simulink model "REGISTROS_64_BITS_02"  (R2022a)
settings: Solver=VariableStepAuto  StartTime=0.0  StopTime=10.0  RelTol=1e-3
undefined symbols (not defined in the file or in its folder): xc7z010iclg225
libraries: hdlBasic x6609, vmcUtilities x1
(part 17 of 23)

== system REGISTROS_64_BITS_02/REGISTRO_64_BITS_8 ==
  D (64 BIT) : Inport
  C - ENABLE (1 BIT) : Inport  Port=2
  Concat1 : hdlBasic/Concat  num_inputs=2  XmcBlockStatus=1  maskContainerNames=group1  block_type=concat  block_config=sysgen:Concat_config
  Convert32 : hdlBasic/Convert  gui_display_data_type=Boolean  arith_type=Boolean  n_bits=16  bin_pt=14  float_type=Single  exp_bits=8  fraction_bits=24  quantization=Truncate  overflow=Wrap  en=off  latency=0  pipeline=off  XmcBlockStatus=1  maskContainerNames=group2  block_type=convert  block_config=sysgen:Convert_config  block_width=595  block_height=885
  D_0 : hdlBasic/Slice  nbits=1  boolean_output=off  mode=Lower Bit Location + Width  bit1=-3  base1=MSB of Input  bit0=0  base0=LSB of Input  XmcBlockStatus=1  maskContainerNames=group1  block_type=slice  block_config=sysgen:Slice_config
  D_1 : hdlBasic/Slice  nbits=1  boolean_output=off  mode=Lower Bit Location + Width  bit1=-2  base1=MSB of Input  bit0=1  base0=LSB of Input  XmcBlockStatus=1  maskContainerNames=group1  block_type=slice  block_config=sysgen:Slice_config
  D_10 : hdlBasic/Slice  nbits=1  boolean_output=off  mode=Lower Bit Location + Width  bit1=-1  base1=MSB of Input  bit0=10  base0=LSB of Input  XmcBlockStatus=1  maskContainerNames=group1  block_type=slice  block_config=sysgen:Slice_config
  D_11 : hdlBasic/Slice  nbits=1  boolean_output=off  mode=Lower Bit Location + Width  bit1=0  base1=MSB of Input  bit0=11  base0=LSB of Input  XmcBlockStatus=1  maskContainerNames=group1  block_type=slice  block_config=sysgen:Slice_config
  D_12 : hdlBasic/Slice  nbits=1  boolean_output=off  mode=Lower Bit Location + Width  bit1=-3  base1=MSB of Input  bit0=12  base0=LSB of Input  XmcBlockStatus=1  maskContainerNames=group1  block_type=slice  block_config=sysgen:Slice_config
  D_13 : hdlBasic/Slice  nbits=1  boolean_output=off  mode=Lower Bit Location + Width  bit1=-2  base1=MSB of Input  bit0=13  base0=LSB of Input  XmcBlockStatus=1  maskContainerNames=group1  block_type=slice  block_config=sysgen:Slice_config
  D_14 : hdlBasic/Slice  nbits=1  boolean_output=off  mode=Lower Bit Location + Width  bit1=-1  base1=MSB of Input  bit0=14  base0=LSB of Input  XmcBlockStatus=1  maskContainerNames=group1  block_type=slice  block_config=sysgen:Slice_config
  D_15 : hdlBasic/Slice  nbits=1  boolean_output=off  mode=Lower Bit Location + Width  bit1=0  base1=MSB of Input  bit0=15  base0=LSB of Input  XmcBlockStatus=1  maskContainerNames=group1  block_type=slice  block_config=sysgen:Slice_config
  D_16 : hdlBasic/Slice  nbits=1  boolean_output=off  mode=Lower Bit Location + Width  bit1=-3  base1=MSB of Input  bit0=16  base0=LSB of Input  XmcBlockStatus=1  maskContainerNames=group1  block_type=slice  block_config=sysgen:Slice_config
  D_17 : hdlBasic/Slice  nbits=1  boolean_output=off  mode=Lower Bit Location + Width  bit1=-2  base1=MSB of Input  bit0=17  base0=LSB of Input  XmcBlockStatus=1  maskContainerNames=group1  block_type=slice  block_config=sysgen:Slice_config
  D_18 : hdlBasic/Slice  nbits=1  boolean_output=off  mode=Lower Bit Location + Width  bit1=-1  base1=MSB of Input  bit0=18  base0=LSB of Input  XmcBlockStatus=1  maskContainerNames=group1  block_type=slice  block_config=sysgen:Slice_config
  D_19 : hdlBasic/Slice  nbits=1  boolean_output=off  mode=Lower Bit Location + Width  bit1=0  base1=MSB of Input  bit0=19  base0=LSB of Input  XmcBlockStatus=1  maskContainerNames=group1  block_type=slice  block_config=sysgen:Slice_config
  D_2 : hdlBasic/Slice  nbits=1  boolean_output=off  mode=Lower Bit Location + Width  bit1=-1  base1=MSB of Input  bit0=2  base0=LSB of Input  XmcBlockStatus=1  maskContainerNames=group1  block_type=slice  block_config=sysgen:Slice_config
  D_20 : hdlBasic/Slice  nbits=1  boolean_output=off  mode=Lower Bit Location + Width  bit1=-3  base1=MSB of Input  bit0=20  base0=LSB of Input  XmcBlockStatus=1  maskContainerNames=group1  block_type=slice  block_config=sysgen:Slice_config
  D_21 : hdlBasic/Slice  nbits=1  boolean_output=off  mode=Lower Bit Location + Width  bit1=-2  base1=MSB of Input  bit0=21  base0=LSB of Input  XmcBlockStatus=1  maskContainerNames=group1  block_type=slice  block_config=sysgen:Slice_config
  D_22 : hdlBasic/Slice  nbits=1  boolean_output=off  mode=Lower Bit Location + Width  bit1=-1  base1=MSB of Input  bit0=22  base0=LSB of Input  XmcBlockStatus=1  maskContainerNames=group1  block_type=slice  block_config=sysgen:Slice_config
  D_23 : hdlBasic/Slice  nbits=1  boolean_output=off  mode=Lower Bit Location + Width  bit1=0  base1=MSB of Input  bit0=23  base0=LSB of Input  XmcBlockStatus=1  maskContainerNames=group1  block_type=slice  block_config=sysgen:Slice_config
  D_24 : hdlBasic/Slice  nbits=1  boolean_output=off  mode=Lower Bit Location + Width  bit1=-3  base1=MSB of Input  bit0=24  base0=LSB of Input  XmcBlockStatus=1  maskContainerNames=group1  block_type=slice  block_config=sysgen:Slice_config
  D_25 : hdlBasic/Slice  nbits=1  boolean_output=off  mode=Lower Bit Location + Width  bit1=-2  base1=MSB of Input  bit0=25  base0=LSB of Input  XmcBlockStatus=1  maskContainerNames=group1  block_type=slice  block_config=sysgen:Slice_config
  D_26 : hdlBasic/Slice  nbits=1  boolean_output=off  mode=Lower Bit Location + Width  bit1=-1  base1=MSB of Input  bit0=26  base0=LSB of Input  XmcBlockStatus=1  maskContainerNames=group1  block_type=slice  block_config=sysgen:Slice_config
  D_27 : hdlBasic/Slice  nbits=1  boolean_output=off  mode=Lower Bit Location + Width  bit1=0  base1=MSB of Input  bit0=27  base0=LSB of Input  XmcBlockStatus=1  maskContainerNames=group1  block_type=slice  block_config=sysgen:Slice_config
  D_28 : hdlBasic/Slice  nbits=1  boolean_output=off  mode=Lower Bit Location + Width  bit1=-3  base1=MSB of Input  bit0=28  base0=LSB of Input  XmcBlockStatus=1  maskContainerNames=group1  block_type=slice  block_config=sysgen:Slice_config
  D_29 : hdlBasic/Slice  nbits=1  boolean_output=off  mode=Lower Bit Location + Width  bit1=-2  base1=MSB of Input  bit0=29  base0=LSB of Input  XmcBlockStatus=1  maskContainerNames=group1  block_type=slice  block_config=sysgen:Slice_config
  D_3 : hdlBasic/Slice  nbits=1  boolean_output=off  mode=Lower Bit Location + Width  bit1=0  base1=MSB of Input  bit0=3  base0=LSB of Input  XmcBlockStatus=1  maskContainerNames=group1  block_type=slice  block_config=sysgen:Slice_config
  D_30 : hdlBasic/Slice  nbits=1  boolean_output=off  mode=Lower Bit Location + Width  bit1=-1  base1=MSB of Input  bit0=30  base0=LSB of Input  XmcBlockStatus=1  maskContainerNames=group1  block_type=slice  block_config=sysgen:Slice_config
  D_31 : hdlBasic/Slice  nbits=1  boolean_output=off  mode=Lower Bit Location + Width  bit1=0  base1=MSB of Input  bit0=31  base0=LSB of Input  XmcBlockStatus=1  maskContainerNames=group1  block_type=slice  block_config=sysgen:Slice_config
  D_32 : hdlBasic/Slice  nbits=1  boolean_output=off  mode=Lower Bit Location + Width  bit1=-3  base1=MSB of Input  bit0=32  base0=LSB of Input  XmcBlockStatus=1  maskContainerNames=group1  block_type=slice  block_config=sysgen:Slice_config
  D_33 : hdlBasic/Slice  nbits=1  boolean_output=off  mode=Lower Bit Location + Width  bit1=-2  base1=MSB of Input  bit0=33  base0=LSB of Input  XmcBlockStatus=1  maskContainerNames=group1  block_type=slice  block_config=sysgen:Slice_config
  D_34 : hdlBasic/Slice  nbits=1  boolean_output=off  mode=Lower Bit Location + Width  bit1=-1  base1=MSB of Input  bit0=34  base0=LSB of Input  XmcBlockStatus=1  maskContainerNames=group1  block_type=slice  block_config=sysgen:Slice_config
  D_35 : hdlBasic/Slice  nbits=1  boolean_output=off  mode=Lower Bit Location + Width  bit1=0  base1=MSB of Input  bit0=35  base0=LSB of Input  XmcBlockStatus=1  maskContainerNames=group1  block_type=slice  block_config=sysgen:Slice_config
  D_36 : hdlBasic/Slice  nbits=1  boolean_output=off  mode=Lower Bit Location + Width  bit1=-3  base1=MSB of Input  bit0=36  base0=LSB of Input  XmcBlockStatus=1  maskContainerNames=group1  block_type=slice  block_config=sysgen:Slice_config
  D_37 : hdlBasic/Slice  nbits=1  boolean_output=off  mode=Lower Bit Location + Width  bit1=-2  base1=MSB of Input  bit0=37  base0=LSB of Input  XmcBlockStatus=1  maskContainerNames=group1  block_type=slice  block_config=sysgen:Slice_config
  D_38 : hdlBasic/Slice  nbits=1  boolean_output=off  mode=Lower Bit Location + Width  bit1=-1  base1=MSB of Input  bit0=38  base0=LSB of Input  XmcBlockStatus=1  maskContainerNames=group1  block_type=slice  block_config=sysgen:Slice_config
  D_39 : hdlBasic/Slice  nbits=1  boolean_output=off  mode=Lower Bit Location + Width  bit1=0  base1=MSB of Input  bit0=39  base0=LSB of Input  XmcBlockStatus=1  maskContainerNames=group1  block_type=slice  block_config=sysgen:Slice_config
  D_4 : hdlBasic/Slice  nbits=1  boolean_output=off  mode=Lower Bit Location + Width  bit1=-3  base1=MSB of Input  bit0=4  base0=LSB of Input  XmcBlockStatus=1  maskContainerNames=group1  block_type=slice  block_config=sysgen:Slice_config
  D_40 : hdlBasic/Slice  nbits=1  boolean_output=off  mode=Lower Bit Location + Width  bit1=-3  base1=MSB of Input  bit0=40  base0=LSB of Input  XmcBlockStatus=1  maskContainerNames=group1  block_type=slice  block_config=sysgen:Slice_config
  D_41 : hdlBasic/Slice  nbits=1  boolean_output=off  mode=Lower Bit Location + Width  bit1=-2  base1=MSB of Input  bit0=41  base0=LSB of Input  XmcBlockStatus=1  maskContainerNames=group1  block_type=slice  block_config=sysgen:Slice_config
  D_42 : hdlBasic/Slice  nbits=1  boolean_output=off  mode=Lower Bit Location + Width  bit1=-1  base1=MSB of Input  bit0=42  base0=LSB of Input  XmcBlockStatus=1  maskContainerNames=group1  block_type=slice  block_config=sysgen:Slice_config
  D_43 : hdlBasic/Slice  nbits=1  boolean_output=off  mode=Lower Bit Location + Width  bit1=0  base1=MSB of Input  bit0=43  base0=LSB of Input  XmcBlockStatus=1  maskContainerNames=group1  block_type=slice  block_config=sysgen:Slice_config
  D_44 : hdlBasic/Slice  nbits=1  boolean_output=off  mode=Lower Bit Location + Width  bit1=-3  base1=MSB of Input  bit0=44  base0=LSB of Input  XmcBlockStatus=1  maskContainerNames=group1  block_type=slice  block_config=sysgen:Slice_config
  D_45 : hdlBasic/Slice  nbits=1  boolean_output=off  mode=Lower Bit Location + Width  bit1=-2  base1=MSB of Input  bit0=45  base0=LSB of Input  XmcBlockStatus=1  maskContainerNames=group1  block_type=slice  block_config=sysgen:Slice_config
  D_46 : hdlBasic/Slice  nbits=1  boolean_output=off  mode=Lower Bit Location + Width  bit1=-1  base1=MSB of Input  bit0=46  base0=LSB of Input  XmcBlockStatus=1  maskContainerNames=group1  block_type=slice  block_config=sysgen:Slice_config
  D_47 : hdlBasic/Slice  nbits=1  boolean_output=off  mode=Lower Bit Location + Width  bit1=0  base1=MSB of Input  bit0=47  base0=LSB of Input  XmcBlockStatus=1  maskContainerNames=group1  block_type=slice  block_config=sysgen:Slice_config
  D_48 : hdlBasic/Slice  nbits=1  boolean_output=off  mode=Lower Bit Location + Width  bit1=-3  base1=MSB of Input  bit0=48  base0=LSB of Input  XmcBlockStatus=1  maskContainerNames=group1  block_type=slice  block_config=sysgen:Slice_config
  D_49 : hdlBasic/Slice  nbits=1  boolean_output=off  mode=Lower Bit Location + Width  bit1=-2  base1=MSB of Input  bit0=49  base0=LSB of Input  XmcBlockStatus=1  maskContainerNames=group1  block_type=slice  block_config=sysgen:Slice_config
  D_5 : hdlBasic/Slice  nbits=1  boolean_output=off  mode=Lower Bit Location + Width  bit1=-2  base1=MSB of Input  bit0=5  base0=LSB of Input  XmcBlockStatus=1  maskContainerNames=group1  block_type=slice  block_config=sysgen:Slice_config
  D_50 : hdlBasic/Slice  nbits=1  boolean_output=off  mode=Lower Bit Location + Width  bit1=-1  base1=MSB of Input  bit0=50  base0=LSB of Input  XmcBlockStatus=1  maskContainerNames=group1  block_type=slice  block_config=sysgen:Slice_config
  D_51 : hdlBasic/Slice  nbits=1  boolean_output=off  mode=Lower Bit Location + Width  bit1=0  base1=MSB of Input  bit0=51  base0=LSB of Input  XmcBlockStatus=1  maskContainerNames=group1  block_type=slice  block_config=sysgen:Slice_config
  D_52 : hdlBasic/Slice  nbits=1  boolean_output=off  mode=Lower Bit Location + Width  bit1=-3  base1=MSB of Input  bit0=52  base0=LSB of Input  XmcBlockStatus=1  maskContainerNames=group1  block_type=slice  block_config=sysgen:Slice_config
  D_53 : hdlBasic/Slice  nbits=1  boolean_output=off  mode=Lower Bit Location + Width  bit1=-2  base1=MSB of Input  bit0=53  base0=LSB of Input  XmcBlockStatus=1  maskContainerNames=group1  block_type=slice  block_config=sysgen:Slice_config
  D_54 : hdlBasic/Slice  nbits=1  boolean_output=off  mode=Lower Bit Location + Width  bit1=-1  base1=MSB of Input  bit0=54  base0=LSB of Input  XmcBlockStatus=1  maskContainerNames=group1  block_type=slice  block_config=sysgen:Slice_config
  D_55 : hdlBasic/Slice  nbits=1  boolean_output=off  mode=Lower Bit Location + Width  bit1=0  base1=MSB of Input  bit0=55  base0=LSB of Input  XmcBlockStatus=1  maskContainerNames=group1  block_type=slice  block_config=sysgen:Slice_config
  D_56 : hdlBasic/Slice  nbits=1  boolean_output=off  mode=Lower Bit Location + Width  bit1=-3  base1=MSB of Input  bit0=56  base0=LSB of Input  XmcBlockStatus=1  maskContainerNames=group1  block_type=slice  block_config=sysgen:Slice_config
  D_57 : hdlBasic/Slice  nbits=1  boolean_output=off  mode=Lower Bit Location + Width  bit1=-2  base1=MSB of Input  bit0=57  base0=LSB of Input  XmcBlockStatus=1  maskContainerNames=group1  block_type=slice  block_config=sysgen:Slice_config
  D_58 : hdlBasic/Slice  nbits=1  boolean_output=off  mode=Lower Bit Location + Width  bit1=-1  base1=MSB of Input  bit0=58  base0=LSB of Input  XmcBlockStatus=1  maskContainerNames=group1  block_type=slice  block_config=sysgen:Slice_config
  D_59 : hdlBasic/Slice  nbits=1  boolean_output=off  mode=Lower Bit Location + Width  bit1=0  base1=MSB of Input  bit0=59  base0=LSB of Input  XmcBlockStatus=1  maskContainerNames=group1  block_type=slice  block_config=sysgen:Slice_config
  D_6 : hdlBasic/Slice  nbits=1  boolean_output=off  mode=Lower Bit Location + Width  bit1=-1  base1=MSB of Input  bit0=6  base0=LSB of Input  XmcBlockStatus=1  maskContainerNames=group1  block_type=slice  block_config=sysgen:Slice_config
  D_60 : hdlBasic/Slice  nbits=1  boolean_output=off  mode=Lower Bit Location + Width  bit1=-3  base1=MSB of Input  bit0=60  base0=LSB of Input  XmcBlockStatus=1  maskContainerNames=group1  block_type=slice  block_config=sysgen:Slice_config
  D_61 : hdlBasic/Slice  nbits=1  boolean_output=off  mode=Lower Bit Location + Width  bit1=-2  base1=MSB of Input  bit0=61  base0=LSB of Input  XmcBlockStatus=1  maskContainerNames=group1  block_type=slice  block_config=sysgen:Slice_config
  D_62 : hdlBasic/Slice  nbits=1  boolean_output=off  mode=Lower Bit Location + Width  bit1=-1  base1=MSB of Input  bit0=62  base0=LSB of Input  XmcBlockStatus=1  maskContainerNames=group1  block_type=slice  block_config=sysgen:Slice_config
  D_63 : hdlBasic/Slice  nbits=1  boolean_output=off  mode=Lower Bit Location + Width  bit1=0  base1=MSB of Input  bit0=63  base0=LSB of Input  XmcBlockStatus=1  maskContainerNames=group1  block_type=slice  block_config=sysgen:Slice_config
  D_7 : hdlBasic/Slice  nbits=1  boolean_output=off  mode=Lower Bit Location + Width  bit1=0  base1=MSB of Input  bit0=7  base0=LSB of Input  XmcBlockStatus=1  maskContainerNames=group1  block_type=slice  block_config=sysgen:Slice_config
  D_8 : hdlBasic/Slice  nbits=1  boolean_output=off  mode=Lower Bit Location + Width  bit1=-3  base1=MSB of Input  bit0=8  base0=LSB of Input  XmcBlockStatus=1  maskContainerNames=group1  block_type=slice  block_config=sysgen:Slice_config
  D_9 : hdlBasic/Slice  nbits=1  boolean_output=off  mode=Lower Bit Location + Width  bit1=-2  base1=MSB of Input  bit0=9  base0=LSB of Input  XmcBlockStatus=1  maskContainerNames=group1  block_type=slice  block_config=sysgen:Slice_config
  Q_OUT_32_BIT1 : Subsystem
  Q_OUT_32_BIT2 : Subsystem
  Register_{1..64} (64 alike) : hdlBasic/Register  init=0  rst=off  en=on  XmcBlockStatus=1  maskContainerNames=tabcontainer1  block_type=register  block_config=sysgen:Register_config
  Q (64 BIT) : Outport
  wires:
  D (64 BIT)/1 -> D_63/1, D_62/1, D_61/1, D_60/1, D_59/1, D_58/1, D_57/1, D_56/1, D_55/1, D_54/1, D_53/1, D_52/1, D_51/1, D_50/1, D_49/1, D_48/1, D_47/1, D_46/1, D_45/1, D_44/1, D_43/1, D_42/1, D_41/1, D_40/1, D_39/1, D_38/1, D_37/1, D_36/1, D_35/1, D_34/1, D_33/1, D_32/1, D_31/1, D_30/1, D_29/1, D_28/1, D_27/1, D_26/1, D_25/1, D_24/1, D_23/1, D_22/1, D_21/1, D_20/1, D_19/1, D_18/1, D_17/1, D_16/1, D_15/1, D_14/1, D_13/1, D_12/1, D_11/1, D_10/1, D_9/1, D_8/1, D_7/1, D_6/1, D_5/1, D_4/1, D_3/1, D_2/1, D_1/1, D_0/1
  Register_27/1 -> Q_OUT_32_BIT2/27(Q_OUT_26 (1 BIT))
  D_59/1 -> Register_28/1
  Register_4/1 -> Q_OUT_32_BIT2/4(Q_OUT_3 (1 BIT))
  Register_21/1 -> Q_OUT_32_BIT2/21(Q_OUT_20 (1 BIT))
  Register_56/1 -> Q_OUT_32_BIT1/25(Q_OUT_24 (1 BIT))
  C - ENABLE (1 BIT)/1 -> Convert32/1
  Register_3/1 -> Q_OUT_32_BIT2/3(Q_OUT_2 (1 BIT))
  D_19/1 -> Register_51/1
  D_12/1 -> Register_44/1
  Convert32/1 -> Register_35/2, Register_49/2, Register_64/2, Register_31/2, Register_30/2, Register_29/2, Register_28/2, Register_27/2, Register_26/2, Register_25/2, Register_24/2, Register_23/2, Register_22/2, Register_21/2, Register_20/2, Register_19/2, Register_18/2, Register_17/2, Register_16/2, Register_15/2, Register_14/2, Register_13/2, Register_12/2, Register_11/2, Register_10/2, Register_9/2, Register_8/2, Register_7/2, Register_6/2, Register_5/2, Register_4/2, Register_3/2, Register_2/2, Register_1/2, Register_63/2, Register_62/2, Register_61/2, Register_60/2, Register_59/2, Register_58/2, Register_57/2, Register_56/2, Register_55/2, Register_54/2, Register_53/2, Register_52/2, Register_51/2, Register_50/2, Register_48/2, Register_47/2, Register_46/2, Register_45/2, Register_44/2, Register_43/2, Register_42/2, Register_41/2, Register_40/2, Register_39/2, Register_38/2, Register_37/2, Register_36/2, Register_34/2, Register_33/2, Register_32/2
  D_2/1 -> Register_34/1
  Register_49/1 -> Q_OUT_32_BIT1/18(Q_OUT_17 (1 BIT))
  D_37/1 -> Register_6/1
  D_3/1 -> Register_35/1
  Register_8/1 -> Q_OUT_32_BIT2/8(Q_OUT_7 (1 BIT))
  D_47/1 -> Register_16/1
  Register_34/1 -> Q_OUT_32_BIT1/3(Q_OUT_2 (1 BIT))
  D_29/1 -> Register_61/1
  Register_26/1 -> Q_OUT_32_BIT2/26(Q_OUT_25 (1 BIT))
  D_6/1 -> Register_38/1
  Register_40/1 -> Q_OUT_32_BIT1/9(Q_OUT_8 (1 BIT))
  D_17/1 -> Register_49/1
  Register_9/1 -> Q_OUT_32_BIT2/9(Q_OUT_8 (1 BIT))
  Register_61/1 -> Q_OUT_32_BIT1/30(Q_OUT_29 (1 BIT))
  D_49/1 -> Register_18/1
  D_32/1 -> Register_1/1
  D_10/1 -> Register_42/1
  Register_62/1 -> Q_OUT_32_BIT1/31(Q_OUT_30 (1 BIT))
  D_18/1 -> Register_50/1
  Register_11/1 -> Q_OUT_32_BIT2/11(Q_OUT_10 (1 BIT))
  D_61/1 -> Register_30/1
  D_16/1 -> Register_48/1
  D_56/1 -> Register_25/1
  Register_30/1 -> Q_OUT_32_BIT2/30(Q_OUT_29 (1 BIT))
  Register_23/1 -> Q_OUT_32_BIT2/23(Q_OUT_22 (1 BIT))
  Concat1/1 -> Q (64 BIT)/1
  D_27/1 -> Register_59/1
  D_1/1 -> Register_33/1
  Register_60/1 -> Q_OUT_32_BIT1/29(Q_OUT_28 (1 BIT))
  Register_59/1 -> Q_OUT_32_BIT1/28(Q_OUT_27 (1 BIT))
  Register_33/1 -> Q_OUT_32_BIT1/2(Q_OUT_1 (1 BIT))
  Register_1/1 -> Q_OUT_32_BIT2/1(Q_OUT_0 (1 BIT))
  Register_5/1 -> Q_OUT_32_BIT2/5(Q_OUT_4 (1 BIT))
  Register_48/1 -> Q_OUT_32_BIT1/17(Q_OUT_16 (1 BIT))
  Register_53/1 -> Q_OUT_32_BIT1/22(Q_OUT_21 (1 BIT))
  D_58/1 -> Register_27/1
  Register_15/1 -> Q_OUT_32_BIT2/15(Q_OUT_14 (1 BIT))
  Register_35/1 -> Q_OUT_32_BIT1/4(Q_OUT_3 (1 BIT))
  D_26/1 -> Register_58/1
  D_22/1 -> Register_54/1
  D_4/1 -> Register_36/1
  D_0/1 -> Register_32/1
  D_23/1 -> Register_55/1
  Register_38/1 -> Q_OUT_32_BIT1/7(Q_OUT_6 (1 BIT))
  D_25/1 -> Register_57/1
  Register_24/1 -> Q_OUT_32_BIT2/24(Q_OUT_23 (1 BIT))
  Register_55/1 -> Q_OUT_32_BIT1/24(Q_OUT_23 (1 BIT))
  Register_16/1 -> Q_OUT_32_BIT2/16(Q_OUT_15 (1 BIT))
  Register_51/1 -> Q_OUT_32_BIT1/20(Q_OUT_19 (1 BIT))
  Register_39/1 -> Q_OUT_32_BIT1/8(Q_OUT_7 (1 BIT))
  Register_42/1 -> Q_OUT_32_BIT1/11(Q_OUT_10 (1 BIT))
  D_38/1 -> Register_7/1
  Register_25/1 -> Q_OUT_32_BIT2/25(Q_OUT_24 (1 BIT))
  D_30/1 -> Register_62/1
  D_53/1 -> Register_22/1
  D_5/1 -> Register_37/1
  D_8/1 -> Register_40/1
  D_11/1 -> Register_43/1
  Register_57/1 -> Q_OUT_32_BIT1/26(Q_OUT_25 (1 BIT))
  Register_54/1 -> Q_OUT_32_BIT1/23(Q_OUT_22 (1 BIT))
  Register_50/1 -> Q_OUT_32_BIT1/19(Q_OUT_18 (1 BIT))
  Register_52/1 -> Q_OUT_32_BIT1/21(Q_OUT_20 (1 BIT))
  Register_44/1 -> Q_OUT_32_BIT1/13(Q_OUT_12 (1 BIT))
  Register_6/1 -> Q_OUT_32_BIT2/6(Q_OUT_5 (1 BIT))
  Register_13/1 -> Q_OUT_32_BIT2/13(Q_OUT_12 (1 BIT))
  D_42/1 -> Register_11/1
  Register_45/1 -> Q_OUT_32_BIT1/14(Q_OUT_13 (1 BIT))
  Register_58/1 -> Q_OUT_32_BIT1/27(Q_OUT_26 (1 BIT))
  Register_64/1 -> Q_OUT_32_BIT2/32(Q_OUT_31 (1 BIT))
  Register_2/1 -> Q_OUT_32_BIT2/2(Q_OUT_1 (1 BIT))
  Register_18/1 -> Q_OUT_32_BIT2/18(Q_OUT_17 (1 BIT))
  Register_31/1 -> Q_OUT_32_BIT2/31(Q_OUT_30 (1 BIT))
  Register_29/1 -> Q_OUT_32_BIT2/29(Q_OUT_28 (1 BIT))
  Register_12/1 -> Q_OUT_32_BIT2/12(Q_OUT_11 (1 BIT))
  Register_14/1 -> Q_OUT_32_BIT2/14(Q_OUT_13 (1 BIT))
  Register_36/1 -> Q_OUT_32_BIT1/5(Q_OUT_4 (1 BIT))
  Register_47/1 -> Q_OUT_32_BIT1/16(Q_OUT_15 (1 BIT))
  Register_41/1 -> Q_OUT_32_BIT1/10(Q_OUT_9 (1 BIT))
  Register_46/1 -> Q_OUT_32_BIT1/15(Q_OUT_14 (1 BIT))
  Register_32/1 -> Q_OUT_32_BIT1/1(Q_OUT_0 (1 BIT))
  D_28/1 -> Register_60/1
  Q_OUT_32_BIT2/1(Q (32 BIT)) -> Concat1/1
  Q_OUT_32_BIT1/1(Q (32 BIT)) -> Concat1/2
  D_43/1 -> Register_12/1
  D_57/1 -> Register_26/1
  D_63/1 -> Register_64/1
  D_45/1 -> Register_14/1
  D_46/1 -> Register_15/1
  D_39/1 -> Register_8/1
  D_52/1 -> Register_21/1
  D_41/1 -> Register_10/1
  D_60/1 -> Register_29/1
  D_35/1 -> Register_4/1
  D_54/1 -> Register_23/1
  D_62/1 -> Register_31/1
  D_15/1 -> Register_47/1
  D_48/1 -> Register_17/1
  D_40/1 -> Register_9/1
  D_7/1 -> Register_39/1
  D_36/1 -> Register_5/1
  D_55/1 -> Register_24/1
  D_51/1 -> Register_20/1
  D_44/1 -> Register_13/1
  D_34/1 -> Register_3/1
  D_33/1 -> Register_2/1
  D_50/1 -> Register_19/1
  D_9/1 -> Register_41/1
  Register_28/1 -> Q_OUT_32_BIT2/28(Q_OUT_27 (1 BIT))
  D_14/1 -> Register_46/1
  Register_7/1 -> Q_OUT_32_BIT2/7(Q_OUT_6 (1 BIT))
  Register_10/1 -> Q_OUT_32_BIT2/10(Q_OUT_9 (1 BIT))
  D_13/1 -> Register_45/1
  D_24/1 -> Register_56/1
  D_31/1 -> Register_63/1
  D_20/1 -> Register_52/1
  D_21/1 -> Register_53/1
  Register_63/1 -> Q_OUT_32_BIT1/32(Q_OUT_31 (1 BIT))
  Register_37/1 -> Q_OUT_32_BIT1/6(Q_OUT_5 (1 BIT))
  Register_20/1 -> Q_OUT_32_BIT2/20(Q_OUT_19 (1 BIT))
  Register_22/1 -> Q_OUT_32_BIT2/22(Q_OUT_21 (1 BIT))
  Register_19/1 -> Q_OUT_32_BIT2/19(Q_OUT_18 (1 BIT))
  Register_17/1 -> Q_OUT_32_BIT2/17(Q_OUT_16 (1 BIT))
  Register_43/1 -> Q_OUT_32_BIT1/12(Q_OUT_11 (1 BIT))

== system REGISTROS_64_BITS_02/REGISTRO_64_BITS_9 ==
  D (64 BIT) : Inport
  C - ENABLE (1 BIT) : Inport  Port=2
  Concat1 : hdlBasic/Concat  num_inputs=2  XmcBlockStatus=1  maskContainerNames=group1  block_type=concat  block_config=sysgen:Concat_config
  Convert32 : hdlBasic/Convert  gui_display_data_type=Boolean  arith_type=Boolean  n_bits=16  bin_pt=14  float_type=Single  exp_bits=8  fraction_bits=24  quantization=Truncate  overflow=Wrap  en=off  latency=0  pipeline=off  XmcBlockStatus=1  maskContainerNames=group2  block_type=convert  block_config=sysgen:Convert_config  block_width=595  block_height=885
  D_0 : hdlBasic/Slice  nbits=1  boolean_output=off  mode=Lower Bit Location + Width  bit1=-3  base1=MSB of Input  bit0=0  base0=LSB of Input  XmcBlockStatus=1  maskContainerNames=group1  block_type=slice  block_config=sysgen:Slice_config
  D_1 : hdlBasic/Slice  nbits=1  boolean_output=off  mode=Lower Bit Location + Width  bit1=-2  base1=MSB of Input  bit0=1  base0=LSB of Input  XmcBlockStatus=1  maskContainerNames=group1  block_type=slice  block_config=sysgen:Slice_config
  D_10 : hdlBasic/Slice  nbits=1  boolean_output=off  mode=Lower Bit Location + Width  bit1=-1  base1=MSB of Input  bit0=10  base0=LSB of Input  XmcBlockStatus=1  maskContainerNames=group1  block_type=slice  block_config=sysgen:Slice_config
  D_11 : hdlBasic/Slice  nbits=1  boolean_output=off  mode=Lower Bit Location + Width  bit1=0  base1=MSB of Input  bit0=11  base0=LSB of Input  XmcBlockStatus=1  maskContainerNames=group1  block_type=slice  block_config=sysgen:Slice_config
  D_12 : hdlBasic/Slice  nbits=1  boolean_output=off  mode=Lower Bit Location + Width  bit1=-3  base1=MSB of Input  bit0=12  base0=LSB of Input  XmcBlockStatus=1  maskContainerNames=group1  block_type=slice  block_config=sysgen:Slice_config
  D_13 : hdlBasic/Slice  nbits=1  boolean_output=off  mode=Lower Bit Location + Width  bit1=-2  base1=MSB of Input  bit0=13  base0=LSB of Input  XmcBlockStatus=1  maskContainerNames=group1  block_type=slice  block_config=sysgen:Slice_config
  D_14 : hdlBasic/Slice  nbits=1  boolean_output=off  mode=Lower Bit Location + Width  bit1=-1  base1=MSB of Input  bit0=14  base0=LSB of Input  XmcBlockStatus=1  maskContainerNames=group1  block_type=slice  block_config=sysgen:Slice_config
  D_15 : hdlBasic/Slice  nbits=1  boolean_output=off  mode=Lower Bit Location + Width  bit1=0  base1=MSB of Input  bit0=15  base0=LSB of Input  XmcBlockStatus=1  maskContainerNames=group1  block_type=slice  block_config=sysgen:Slice_config
  D_16 : hdlBasic/Slice  nbits=1  boolean_output=off  mode=Lower Bit Location + Width  bit1=-3  base1=MSB of Input  bit0=16  base0=LSB of Input  XmcBlockStatus=1  maskContainerNames=group1  block_type=slice  block_config=sysgen:Slice_config
  D_17 : hdlBasic/Slice  nbits=1  boolean_output=off  mode=Lower Bit Location + Width  bit1=-2  base1=MSB of Input  bit0=17  base0=LSB of Input  XmcBlockStatus=1  maskContainerNames=group1  block_type=slice  block_config=sysgen:Slice_config
  D_18 : hdlBasic/Slice  nbits=1  boolean_output=off  mode=Lower Bit Location + Width  bit1=-1  base1=MSB of Input  bit0=18  base0=LSB of Input  XmcBlockStatus=1  maskContainerNames=group1  block_type=slice  block_config=sysgen:Slice_config
  D_19 : hdlBasic/Slice  nbits=1  boolean_output=off  mode=Lower Bit Location + Width  bit1=0  base1=MSB of Input  bit0=19  base0=LSB of Input  XmcBlockStatus=1  maskContainerNames=group1  block_type=slice  block_config=sysgen:Slice_config
  D_2 : hdlBasic/Slice  nbits=1  boolean_output=off  mode=Lower Bit Location + Width  bit1=-1  base1=MSB of Input  bit0=2  base0=LSB of Input  XmcBlockStatus=1  maskContainerNames=group1  block_type=slice  block_config=sysgen:Slice_config
  D_20 : hdlBasic/Slice  nbits=1  boolean_output=off  mode=Lower Bit Location + Width  bit1=-3  base1=MSB of Input  bit0=20  base0=LSB of Input  XmcBlockStatus=1  maskContainerNames=group1  block_type=slice  block_config=sysgen:Slice_config
  D_21 : hdlBasic/Slice  nbits=1  boolean_output=off  mode=Lower Bit Location + Width  bit1=-2  base1=MSB of Input  bit0=21  base0=LSB of Input  XmcBlockStatus=1  maskContainerNames=group1  block_type=slice  block_config=sysgen:Slice_config
  D_22 : hdlBasic/Slice  nbits=1  boolean_output=off  mode=Lower Bit Location + Width  bit1=-1  base1=MSB of Input  bit0=22  base0=LSB of Input  XmcBlockStatus=1  maskContainerNames=group1  block_type=slice  block_config=sysgen:Slice_config
  D_23 : hdlBasic/Slice  nbits=1  boolean_output=off  mode=Lower Bit Location + Width  bit1=0  base1=MSB of Input  bit0=23  base0=LSB of Input  XmcBlockStatus=1  maskContainerNames=group1  block_type=slice  block_config=sysgen:Slice_config
  D_24 : hdlBasic/Slice  nbits=1  boolean_output=off  mode=Lower Bit Location + Width  bit1=-3  base1=MSB of Input  bit0=24  base0=LSB of Input  XmcBlockStatus=1  maskContainerNames=group1  block_type=slice  block_config=sysgen:Slice_config
  D_25 : hdlBasic/Slice  nbits=1  boolean_output=off  mode=Lower Bit Location + Width  bit1=-2  base1=MSB of Input  bit0=25  base0=LSB of Input  XmcBlockStatus=1  maskContainerNames=group1  block_type=slice  block_config=sysgen:Slice_config
  D_26 : hdlBasic/Slice  nbits=1  boolean_output=off  mode=Lower Bit Location + Width  bit1=-1  base1=MSB of Input  bit0=26  base0=LSB of Input  XmcBlockStatus=1  maskContainerNames=group1  block_type=slice  block_config=sysgen:Slice_config
  D_27 : hdlBasic/Slice  nbits=1  boolean_output=off  mode=Lower Bit Location + Width  bit1=0  base1=MSB of Input  bit0=27  base0=LSB of Input  XmcBlockStatus=1  maskContainerNames=group1  block_type=slice  block_config=sysgen:Slice_config
  D_28 : hdlBasic/Slice  nbits=1  boolean_output=off  mode=Lower Bit Location + Width  bit1=-3  base1=MSB of Input  bit0=28  base0=LSB of Input  XmcBlockStatus=1  maskContainerNames=group1  block_type=slice  block_config=sysgen:Slice_config
  D_29 : hdlBasic/Slice  nbits=1  boolean_output=off  mode=Lower Bit Location + Width  bit1=-2  base1=MSB of Input  bit0=29  base0=LSB of Input  XmcBlockStatus=1  maskContainerNames=group1  block_type=slice  block_config=sysgen:Slice_config
  D_3 : hdlBasic/Slice  nbits=1  boolean_output=off  mode=Lower Bit Location + Width  bit1=0  base1=MSB of Input  bit0=3  base0=LSB of Input  XmcBlockStatus=1  maskContainerNames=group1  block_type=slice  block_config=sysgen:Slice_config
  D_30 : hdlBasic/Slice  nbits=1  boolean_output=off  mode=Lower Bit Location + Width  bit1=-1  base1=MSB of Input  bit0=30  base0=LSB of Input  XmcBlockStatus=1  maskContainerNames=group1  block_type=slice  block_config=sysgen:Slice_config
  D_31 : hdlBasic/Slice  nbits=1  boolean_output=off  mode=Lower Bit Location + Width  bit1=0  base1=MSB of Input  bit0=31  base0=LSB of Input  XmcBlockStatus=1  maskContainerNames=group1  block_type=slice  block_config=sysgen:Slice_config
  D_32 : hdlBasic/Slice  nbits=1  boolean_output=off  mode=Lower Bit Location + Width  bit1=-3  base1=MSB of Input  bit0=32  base0=LSB of Input  XmcBlockStatus=1  maskContainerNames=group1  block_type=slice  block_config=sysgen:Slice_config
  D_33 : hdlBasic/Slice  nbits=1  boolean_output=off  mode=Lower Bit Location + Width  bit1=-2  base1=MSB of Input  bit0=33  base0=LSB of Input  XmcBlockStatus=1  maskContainerNames=group1  block_type=slice  block_config=sysgen:Slice_config
  D_34 : hdlBasic/Slice  nbits=1  boolean_output=off  mode=Lower Bit Location + Width  bit1=-1  base1=MSB of Input  bit0=34  base0=LSB of Input  XmcBlockStatus=1  maskContainerNames=group1  block_type=slice  block_config=sysgen:Slice_config
  D_35 : hdlBasic/Slice  nbits=1  boolean_output=off  mode=Lower Bit Location + Width  bit1=0  base1=MSB of Input  bit0=35  base0=LSB of Input  XmcBlockStatus=1  maskContainerNames=group1  block_type=slice  block_config=sysgen:Slice_config
  D_36 : hdlBasic/Slice  nbits=1  boolean_output=off  mode=Lower Bit Location + Width  bit1=-3  base1=MSB of Input  bit0=36  base0=LSB of Input  XmcBlockStatus=1  maskContainerNames=group1  block_type=slice  block_config=sysgen:Slice_config
  D_37 : hdlBasic/Slice  nbits=1  boolean_output=off  mode=Lower Bit Location + Width  bit1=-2  base1=MSB of Input  bit0=37  base0=LSB of Input  XmcBlockStatus=1  maskContainerNames=group1  block_type=slice  block_config=sysgen:Slice_config
  D_38 : hdlBasic/Slice  nbits=1  boolean_output=off  mode=Lower Bit Location + Width  bit1=-1  base1=MSB of Input  bit0=38  base0=LSB of Input  XmcBlockStatus=1  maskContainerNames=group1  block_type=slice  block_config=sysgen:Slice_config
  D_39 : hdlBasic/Slice  nbits=1  boolean_output=off  mode=Lower Bit Location + Width  bit1=0  base1=MSB of Input  bit0=39  base0=LSB of Input  XmcBlockStatus=1  maskContainerNames=group1  block_type=slice  block_config=sysgen:Slice_config
  D_4 : hdlBasic/Slice  nbits=1  boolean_output=off  mode=Lower Bit Location + Width  bit1=-3  base1=MSB of Input  bit0=4  base0=LSB of Input  XmcBlockStatus=1  maskContainerNames=group1  block_type=slice  block_config=sysgen:Slice_config
  D_40 : hdlBasic/Slice  nbits=1  boolean_output=off  mode=Lower Bit Location + Width  bit1=-3  base1=MSB of Input  bit0=40  base0=LSB of Input  XmcBlockStatus=1  maskContainerNames=group1  block_type=slice  block_config=sysgen:Slice_config
  D_41 : hdlBasic/Slice  nbits=1  boolean_output=off  mode=Lower Bit Location + Width  bit1=-2  base1=MSB of Input  bit0=41  base0=LSB of Input  XmcBlockStatus=1  maskContainerNames=group1  block_type=slice  block_config=sysgen:Slice_config
  D_42 : hdlBasic/Slice  nbits=1  boolean_output=off  mode=Lower Bit Location + Width  bit1=-1  base1=MSB of Input  bit0=42  base0=LSB of Input  XmcBlockStatus=1  maskContainerNames=group1  block_type=slice  block_config=sysgen:Slice_config
  D_43 : hdlBasic/Slice  nbits=1  boolean_output=off  mode=Lower Bit Location + Width  bit1=0  base1=MSB of Input  bit0=43  base0=LSB of Input  XmcBlockStatus=1  maskContainerNames=group1  block_type=slice  block_config=sysgen:Slice_config
  D_44 : hdlBasic/Slice  nbits=1  boolean_output=off  mode=Lower Bit Location + Width  bit1=-3  base1=MSB of Input  bit0=44  base0=LSB of Input  XmcBlockStatus=1  maskContainerNames=group1  block_type=slice  block_config=sysgen:Slice_config
  D_45 : hdlBasic/Slice  nbits=1  boolean_output=off  mode=Lower Bit Location + Width  bit1=-2  base1=MSB of Input  bit0=45  base0=LSB of Input  XmcBlockStatus=1  maskContainerNames=group1  block_type=slice  block_config=sysgen:Slice_config
  D_46 : hdlBasic/Slice  nbits=1  boolean_output=off  mode=Lower Bit Location + Width  bit1=-1  base1=MSB of Input  bit0=46  base0=LSB of Input  XmcBlockStatus=1  maskContainerNames=group1  block_type=slice  block_config=sysgen:Slice_config
  D_47 : hdlBasic/Slice  nbits=1  boolean_output=off  mode=Lower Bit Location + Width  bit1=0  base1=MSB of Input  bit0=47  base0=LSB of Input  XmcBlockStatus=1  maskContainerNames=group1  block_type=slice  block_config=sysgen:Slice_config
  D_48 : hdlBasic/Slice  nbits=1  boolean_output=off  mode=Lower Bit Location + Width  bit1=-3  base1=MSB of Input  bit0=48  base0=LSB of Input  XmcBlockStatus=1  maskContainerNames=group1  block_type=slice  block_config=sysgen:Slice_config
  D_49 : hdlBasic/Slice  nbits=1  boolean_output=off  mode=Lower Bit Location + Width  bit1=-2  base1=MSB of Input  bit0=49  base0=LSB of Input  XmcBlockStatus=1  maskContainerNames=group1  block_type=slice  block_config=sysgen:Slice_config
  D_5 : hdlBasic/Slice  nbits=1  boolean_output=off  mode=Lower Bit Location + Width  bit1=-2  base1=MSB of Input  bit0=5  base0=LSB of Input  XmcBlockStatus=1  maskContainerNames=group1  block_type=slice  block_config=sysgen:Slice_config
  D_50 : hdlBasic/Slice  nbits=1  boolean_output=off  mode=Lower Bit Location + Width  bit1=-1  base1=MSB of Input  bit0=50  base0=LSB of Input  XmcBlockStatus=1  maskContainerNames=group1  block_type=slice  block_config=sysgen:Slice_config
  D_51 : hdlBasic/Slice  nbits=1  boolean_output=off  mode=Lower Bit Location + Width  bit1=0  base1=MSB of Input  bit0=51  base0=LSB of Input  XmcBlockStatus=1  maskContainerNames=group1  block_type=slice  block_config=sysgen:Slice_config
  D_52 : hdlBasic/Slice  nbits=1  boolean_output=off  mode=Lower Bit Location + Width  bit1=-3  base1=MSB of Input  bit0=52  base0=LSB of Input  XmcBlockStatus=1  maskContainerNames=group1  block_type=slice  block_config=sysgen:Slice_config
  D_53 : hdlBasic/Slice  nbits=1  boolean_output=off  mode=Lower Bit Location + Width  bit1=-2  base1=MSB of Input  bit0=53  base0=LSB of Input  XmcBlockStatus=1  maskContainerNames=group1  block_type=slice  block_config=sysgen:Slice_config
  D_54 : hdlBasic/Slice  nbits=1  boolean_output=off  mode=Lower Bit Location + Width  bit1=-1  base1=MSB of Input  bit0=54  base0=LSB of Input  XmcBlockStatus=1  maskContainerNames=group1  block_type=slice  block_config=sysgen:Slice_config
  D_55 : hdlBasic/Slice  nbits=1  boolean_output=off  mode=Lower Bit Location + Width  bit1=0  base1=MSB of Input  bit0=55  base0=LSB of Input  XmcBlockStatus=1  maskContainerNames=group1  block_type=slice  block_config=sysgen:Slice_config
  D_56 : hdlBasic/Slice  nbits=1  boolean_output=off  mode=Lower Bit Location + Width  bit1=-3  base1=MSB of Input  bit0=56  base0=LSB of Input  XmcBlockStatus=1  maskContainerNames=group1  block_type=slice  block_config=sysgen:Slice_config
  D_57 : hdlBasic/Slice  nbits=1  boolean_output=off  mode=Lower Bit Location + Width  bit1=-2  base1=MSB of Input  bit0=57  base0=LSB of Input  XmcBlockStatus=1  maskContainerNames=group1  block_type=slice  block_config=sysgen:Slice_config
  D_58 : hdlBasic/Slice  nbits=1  boolean_output=off  mode=Lower Bit Location + Width  bit1=-1  base1=MSB of Input  bit0=58  base0=LSB of Input  XmcBlockStatus=1  maskContainerNames=group1  block_type=slice  block_config=sysgen:Slice_config
  D_59 : hdlBasic/Slice  nbits=1  boolean_output=off  mode=Lower Bit Location + Width  bit1=0  base1=MSB of Input  bit0=59  base0=LSB of Input  XmcBlockStatus=1  maskContainerNames=group1  block_type=slice  block_config=sysgen:Slice_config
  D_6 : hdlBasic/Slice  nbits=1  boolean_output=off  mode=Lower Bit Location + Width  bit1=-1  base1=MSB of Input  bit0=6  base0=LSB of Input  XmcBlockStatus=1  maskContainerNames=group1  block_type=slice  block_config=sysgen:Slice_config
  D_60 : hdlBasic/Slice  nbits=1  boolean_output=off  mode=Lower Bit Location + Width  bit1=-3  base1=MSB of Input  bit0=60  base0=LSB of Input  XmcBlockStatus=1  maskContainerNames=group1  block_type=slice  block_config=sysgen:Slice_config
  D_61 : hdlBasic/Slice  nbits=1  boolean_output=off  mode=Lower Bit Location + Width  bit1=-2  base1=MSB of Input  bit0=61  base0=LSB of Input  XmcBlockStatus=1  maskContainerNames=group1  block_type=slice  block_config=sysgen:Slice_config
  D_62 : hdlBasic/Slice  nbits=1  boolean_output=off  mode=Lower Bit Location + Width  bit1=-1  base1=MSB of Input  bit0=62  base0=LSB of Input  XmcBlockStatus=1  maskContainerNames=group1  block_type=slice  block_config=sysgen:Slice_config
  D_63 : hdlBasic/Slice  nbits=1  boolean_output=off  mode=Lower Bit Location + Width  bit1=0  base1=MSB of Input  bit0=63  base0=LSB of Input  XmcBlockStatus=1  maskContainerNames=group1  block_type=slice  block_config=sysgen:Slice_config
  D_7 : hdlBasic/Slice  nbits=1  boolean_output=off  mode=Lower Bit Location + Width  bit1=0  base1=MSB of Input  bit0=7  base0=LSB of Input  XmcBlockStatus=1  maskContainerNames=group1  block_type=slice  block_config=sysgen:Slice_config
  D_8 : hdlBasic/Slice  nbits=1  boolean_output=off  mode=Lower Bit Location + Width  bit1=-3  base1=MSB of Input  bit0=8  base0=LSB of Input  XmcBlockStatus=1  maskContainerNames=group1  block_type=slice  block_config=sysgen:Slice_config
  D_9 : hdlBasic/Slice  nbits=1  boolean_output=off  mode=Lower Bit Location + Width  bit1=-2  base1=MSB of Input  bit0=9  base0=LSB of Input  XmcBlockStatus=1  maskContainerNames=group1  block_type=slice  block_config=sysgen:Slice_config
  Q_OUT_32_BIT1 : Subsystem
  Q_OUT_32_BIT2 : Subsystem
  Register_{1..64} (64 alike) : hdlBasic/Register  init=0  rst=off  en=on  XmcBlockStatus=1  maskContainerNames=tabcontainer1  block_type=register  block_config=sysgen:Register_config
  Q (64 BIT) : Outport
  wires:
  D (64 BIT)/1 -> D_63/1, D_62/1, D_61/1, D_60/1, D_59/1, D_58/1, D_57/1, D_56/1, D_55/1, D_54/1, D_53/1, D_52/1, D_51/1, D_50/1, D_49/1, D_48/1, D_47/1, D_46/1, D_45/1, D_44/1, D_43/1, D_42/1, D_41/1, D_40/1, D_39/1, D_38/1, D_37/1, D_36/1, D_35/1, D_34/1, D_33/1, D_32/1, D_31/1, D_30/1, D_29/1, D_28/1, D_27/1, D_26/1, D_25/1, D_24/1, D_23/1, D_22/1, D_21/1, D_20/1, D_19/1, D_18/1, D_17/1, D_16/1, D_15/1, D_14/1, D_13/1, D_12/1, D_11/1, D_10/1, D_9/1, D_8/1, D_7/1, D_6/1, D_5/1, D_4/1, D_3/1, D_2/1, D_1/1, D_0/1
  Register_27/1 -> Q_OUT_32_BIT2/27(Q_OUT_26 (1 BIT))
  D_59/1 -> Register_28/1
  Register_4/1 -> Q_OUT_32_BIT2/4(Q_OUT_3 (1 BIT))
  Register_21/1 -> Q_OUT_32_BIT2/21(Q_OUT_20 (1 BIT))
  Register_56/1 -> Q_OUT_32_BIT1/25(Q_OUT_24 (1 BIT))
  C - ENABLE (1 BIT)/1 -> Convert32/1
  Register_3/1 -> Q_OUT_32_BIT2/3(Q_OUT_2 (1 BIT))
  D_19/1 -> Register_51/1
  D_12/1 -> Register_44/1
  Convert32/1 -> Register_35/2, Register_49/2, Register_64/2, Register_31/2, Register_30/2, Register_29/2, Register_28/2, Register_27/2, Register_26/2, Register_25/2, Register_24/2, Register_23/2, Register_22/2, Register_21/2, Register_20/2, Register_19/2, Register_18/2, Register_17/2, Register_16/2, Register_15/2, Register_14/2, Register_13/2, Register_12/2, Register_11/2, Register_10/2, Register_9/2, Register_8/2, Register_7/2, Register_6/2, Register_5/2, Register_4/2, Register_3/2, Register_2/2, Register_1/2, Register_63/2, Register_62/2, Register_61/2, Register_60/2, Register_59/2, Register_58/2, Register_57/2, Register_56/2, Register_55/2, Register_54/2, Register_53/2, Register_52/2, Register_51/2, Register_50/2, Register_48/2, Register_47/2, Register_46/2, Register_45/2, Register_44/2, Register_43/2, Register_42/2, Register_41/2, Register_40/2, Register_39/2, Register_38/2, Register_37/2, Register_36/2, Register_34/2, Register_33/2, Register_32/2
  D_2/1 -> Register_34/1
  Register_49/1 -> Q_OUT_32_BIT1/18(Q_OUT_17 (1 BIT))
  D_37/1 -> Register_6/1
  D_3/1 -> Register_35/1
  Register_8/1 -> Q_OUT_32_BIT2/8(Q_OUT_7 (1 BIT))
  D_47/1 -> Register_16/1
  Register_34/1 -> Q_OUT_32_BIT1/3(Q_OUT_2 (1 BIT))
  D_29/1 -> Register_61/1
  Register_26/1 -> Q_OUT_32_BIT2/26(Q_OUT_25 (1 BIT))
  D_6/1 -> Register_38/1
  Register_40/1 -> Q_OUT_32_BIT1/9(Q_OUT_8 (1 BIT))
  D_17/1 -> Register_49/1
  Register_9/1 -> Q_OUT_32_BIT2/9(Q_OUT_8 (1 BIT))
  Register_61/1 -> Q_OUT_32_BIT1/30(Q_OUT_29 (1 BIT))
  D_49/1 -> Register_18/1
  D_32/1 -> Register_1/1
  D_10/1 -> Register_42/1
  Register_62/1 -> Q_OUT_32_BIT1/31(Q_OUT_30 (1 BIT))
  D_18/1 -> Register_50/1
  Register_11/1 -> Q_OUT_32_BIT2/11(Q_OUT_10 (1 BIT))
  D_61/1 -> Register_30/1
  D_16/1 -> Register_48/1
  D_56/1 -> Register_25/1
  Register_30/1 -> Q_OUT_32_BIT2/30(Q_OUT_29 (1 BIT))
  Register_23/1 -> Q_OUT_32_BIT2/23(Q_OUT_22 (1 BIT))
  Concat1/1 -> Q (64 BIT)/1
  D_27/1 -> Register_59/1
  D_1/1 -> Register_33/1
  Register_60/1 -> Q_OUT_32_BIT1/29(Q_OUT_28 (1 BIT))
  Register_59/1 -> Q_OUT_32_BIT1/28(Q_OUT_27 (1 BIT))
  Register_33/1 -> Q_OUT_32_BIT1/2(Q_OUT_1 (1 BIT))
  Register_1/1 -> Q_OUT_32_BIT2/1(Q_OUT_0 (1 BIT))
  Register_5/1 -> Q_OUT_32_BIT2/5(Q_OUT_4 (1 BIT))
  Register_48/1 -> Q_OUT_32_BIT1/17(Q_OUT_16 (1 BIT))
  Register_53/1 -> Q_OUT_32_BIT1/22(Q_OUT_21 (1 BIT))
  D_58/1 -> Register_27/1
  Register_15/1 -> Q_OUT_32_BIT2/15(Q_OUT_14 (1 BIT))
  Register_35/1 -> Q_OUT_32_BIT1/4(Q_OUT_3 (1 BIT))
  D_26/1 -> Register_58/1
  D_22/1 -> Register_54/1
  D_4/1 -> Register_36/1
  D_0/1 -> Register_32/1
  D_23/1 -> Register_55/1
  Register_38/1 -> Q_OUT_32_BIT1/7(Q_OUT_6 (1 BIT))
  D_25/1 -> Register_57/1
  Register_24/1 -> Q_OUT_32_BIT2/24(Q_OUT_23 (1 BIT))
  Register_55/1 -> Q_OUT_32_BIT1/24(Q_OUT_23 (1 BIT))
  Register_16/1 -> Q_OUT_32_BIT2/16(Q_OUT_15 (1 BIT))
  Register_51/1 -> Q_OUT_32_BIT1/20(Q_OUT_19 (1 BIT))
  Register_39/1 -> Q_OUT_32_BIT1/8(Q_OUT_7 (1 BIT))
  Register_42/1 -> Q_OUT_32_BIT1/11(Q_OUT_10 (1 BIT))
  D_38/1 -> Register_7/1
  Register_25/1 -> Q_OUT_32_BIT2/25(Q_OUT_24 (1 BIT))
  D_30/1 -> Register_62/1
  D_53/1 -> Register_22/1
  D_5/1 -> Register_37/1
  D_8/1 -> Register_40/1
  D_11/1 -> Register_43/1
  Register_57/1 -> Q_OUT_32_BIT1/26(Q_OUT_25 (1 BIT))
  Register_54/1 -> Q_OUT_32_BIT1/23(Q_OUT_22 (1 BIT))
  Register_50/1 -> Q_OUT_32_BIT1/19(Q_OUT_18 (1 BIT))
  Register_52/1 -> Q_OUT_32_BIT1/21(Q_OUT_20 (1 BIT))
  Register_44/1 -> Q_OUT_32_BIT1/13(Q_OUT_12 (1 BIT))
  Register_6/1 -> Q_OUT_32_BIT2/6(Q_OUT_5 (1 BIT))
  Register_13/1 -> Q_OUT_32_BIT2/13(Q_OUT_12 (1 BIT))
  D_42/1 -> Register_11/1
  Register_45/1 -> Q_OUT_32_BIT1/14(Q_OUT_13 (1 BIT))
  Register_58/1 -> Q_OUT_32_BIT1/27(Q_OUT_26 (1 BIT))
  Register_64/1 -> Q_OUT_32_BIT2/32(Q_OUT_31 (1 BIT))
  Register_2/1 -> Q_OUT_32_BIT2/2(Q_OUT_1 (1 BIT))
  Register_18/1 -> Q_OUT_32_BIT2/18(Q_OUT_17 (1 BIT))
  Register_31/1 -> Q_OUT_32_BIT2/31(Q_OUT_30 (1 BIT))
  Register_29/1 -> Q_OUT_32_BIT2/29(Q_OUT_28 (1 BIT))
  Register_12/1 -> Q_OUT_32_BIT2/12(Q_OUT_11 (1 BIT))
  Register_14/1 -> Q_OUT_32_BIT2/14(Q_OUT_13 (1 BIT))
  Register_36/1 -> Q_OUT_32_BIT1/5(Q_OUT_4 (1 BIT))
  Register_47/1 -> Q_OUT_32_BIT1/16(Q_OUT_15 (1 BIT))
  Register_41/1 -> Q_OUT_32_BIT1/10(Q_OUT_9 (1 BIT))
  Register_46/1 -> Q_OUT_32_BIT1/15(Q_OUT_14 (1 BIT))
  Register_32/1 -> Q_OUT_32_BIT1/1(Q_OUT_0 (1 BIT))
  D_28/1 -> Register_60/1
  Q_OUT_32_BIT2/1(Q (32 BIT)) -> Concat1/1
  Q_OUT_32_BIT1/1(Q (32 BIT)) -> Concat1/2
  D_43/1 -> Register_12/1
  D_57/1 -> Register_26/1
  D_63/1 -> Register_64/1
  D_45/1 -> Register_14/1
  D_46/1 -> Register_15/1
  D_39/1 -> Register_8/1
  D_52/1 -> Register_21/1
  D_41/1 -> Register_10/1
  D_60/1 -> Register_29/1
  D_35/1 -> Register_4/1
  D_54/1 -> Register_23/1
  D_62/1 -> Register_31/1
  D_15/1 -> Register_47/1
  D_48/1 -> Register_17/1
  D_40/1 -> Register_9/1
  D_7/1 -> Register_39/1
  D_36/1 -> Register_5/1
  D_55/1 -> Register_24/1
  D_51/1 -> Register_20/1
  D_44/1 -> Register_13/1
  D_34/1 -> Register_3/1
  D_33/1 -> Register_2/1
  D_50/1 -> Register_19/1
  D_9/1 -> Register_41/1
  Register_28/1 -> Q_OUT_32_BIT2/28(Q_OUT_27 (1 BIT))
  D_14/1 -> Register_46/1
  Register_7/1 -> Q_OUT_32_BIT2/7(Q_OUT_6 (1 BIT))
  Register_10/1 -> Q_OUT_32_BIT2/10(Q_OUT_9 (1 BIT))
  D_13/1 -> Register_45/1
  D_24/1 -> Register_56/1
  D_31/1 -> Register_63/1
  D_20/1 -> Register_52/1
  D_21/1 -> Register_53/1
  Register_63/1 -> Q_OUT_32_BIT1/32(Q_OUT_31 (1 BIT))
  Register_37/1 -> Q_OUT_32_BIT1/6(Q_OUT_5 (1 BIT))
  Register_20/1 -> Q_OUT_32_BIT2/20(Q_OUT_19 (1 BIT))
  Register_22/1 -> Q_OUT_32_BIT2/22(Q_OUT_21 (1 BIT))
  Register_19/1 -> Q_OUT_32_BIT2/19(Q_OUT_18 (1 BIT))
  Register_17/1 -> Q_OUT_32_BIT2/17(Q_OUT_16 (1 BIT))
  Register_43/1 -> Q_OUT_32_BIT1/12(Q_OUT_11 (1 BIT))
